simulink model "Project2FinalModel"  (R2024b)
settings: Solver=VariableStepAuto  StartTime=0.0  StopTime=300  RelTol=1e-3
values from neighbouring files (symbols this model uses):
  ca_f = 60000    [Project2Week1.m]
  ca_r = 90000    [Project2Week1.m]
  omega0 = 0    [Project2Week1.m]
  psi0 = 0    [Project2Week1.m]
  R = 200    [Project2Week1.m]
  vin = 2500    [Project2Week1.m]
  vlf = 1.25    [Project2Week1.m]
  vlr = vwbase - vlf    (= 1.25)    [Project2Week1.m]
  vmass = 1500    [Project2Week1.m]
  vwbase = 2.5    [Project2Week1.m]
  vy0 = 0    [Project2Week1.m]
  X0 = 0    [Project2Week1.m]
  Xd_simulink = [t_waypoints, Xd']    [Project2Week1.m]
  Y0 = 0    [Project2Week1.m]
  Yd_simulink = [t_waypoints, Yd']    [Project2Week1.m]
settings Model: Creator=btagl  LastModifiedBy=btagl

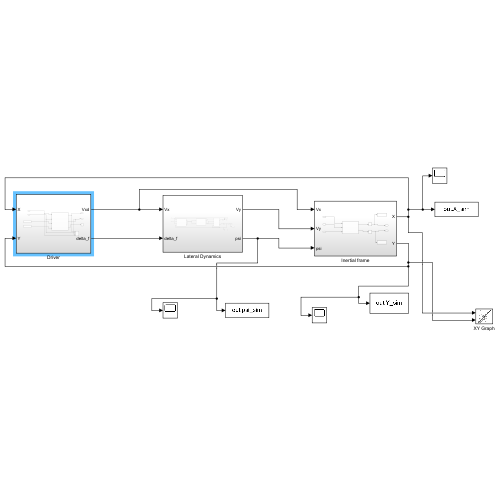
[thumbnail: Simulink's stored preview of the top-level diagram]
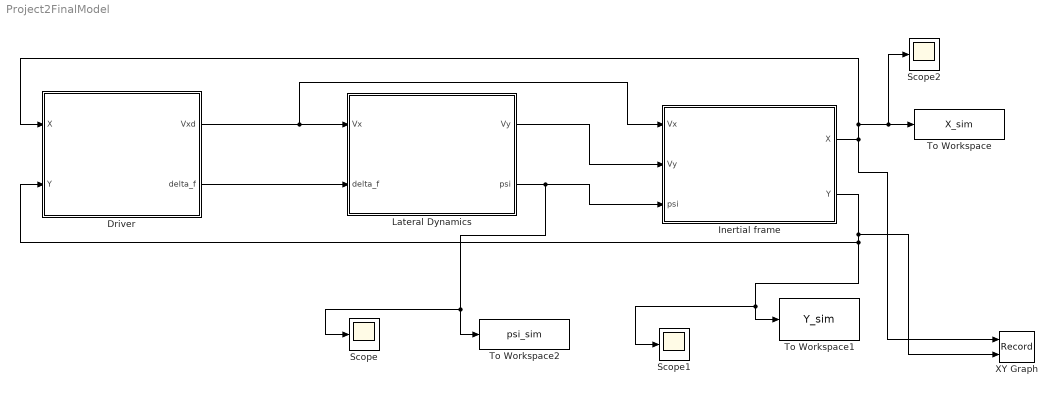
== system Project2FinalModel ==
  Driver : Subsystem
  Inertial frame : Subsystem
  Lateral Dynamics : Subsystem
  Scope : Scope
  Scope1 : Scope
  Scope2 : Scope
  To Workspace : ToWorkspace  VariableName=X_sim  SampleTime=-1
      settings: Save2DSignal=2-D array (concatenate along first dimension)
  To Workspace1 : ToWorkspace  VariableName=Y_sim  SampleTime=-1
      settings: Save2DSignal=2-D array (concatenate along first dimension)
  To Workspace2 : ToWorkspace  VariableName=psi_sim  SampleTime=-1
      settings: Save2DSignal=2-D array (concatenate along first dimension)
  XY Graph : Record  FileSettingsInternal="{\"entries\":[{\"content\":{\"excelSettings\":{\"content\":{},\"type\":\"Streamout.ExcelSettings\"}},\"type\":\"Streamout.FileSettingStorage\",\"uuid\":\"\"}],\"packageUris\":[\"http:\\/\\/schema.mathworks.com\\/mf0\\/streamout_blocks\\/R2020a\"],\"version\":\"1.0\"}"  Layout=[1 1]  SignalsInternal="{\"entries\":[{\"content\":{\"signals\":[{\"content\":{\"blockPath\":[],\"dimensions\":[1],\"domain\":\"\",\"lineColor\":\"#a2142f\",\"plots\":[ 1 ],\"port\":1,\"sid\":[\"\"],\"signalID\":1,\"signalName\":\"Inertial frame:1\"},\"type\":\"RecordBlkView.Signal\",\"uuid\":\"\"},{\"content\":{\"blockPath\":[],\"dimensions\":[1],\"domain\":\"\",\"lineColor\":\"#139fff\",\"plots\":[ 1 ],\"port\":2,\"sid\":[\"\"],\"signalID\":2,\"signalName\":\"Inertial frame:2\"},\"type\":\"RecordBlkView.Signal\",\"uuid\":\"\"}]},\"type\":\"RecordBlkView.InputSignals\",\"uuid\":\"\"}],\"packageUris\":[\"http:\\/\\/schema.mathworks.com\\/mf0\\/streamout_blocks\\/R2020a\"],\"version\":\"1.0\"}"  VisualizationBindings="{\"xyplotplugin\":{\"info\":[{\"series\":[{\"bindingParametersList\":[{\"parameter\":\"X-Axis\",\"signalID\":1,\"signalName\":\"Inertial frame:1\"},{\"parameter\":\"Y-Axis\",\"signalID\":2,\"signalName\":\"Inertial frame:2\"}],\"seriesID\":0}],\"subplotID\":1}]}}"  CompatibilityTag=XY
  wires:
  Driver/1(Vxd) -> Inertial frame/1(Vx), Lateral Dynamics/1(Vx)
  Driver/2(delta_f) -> Lateral Dynamics/2(delta_f)
  Inertial frame/2(Y) -> Scope1/1, To Workspace1/1, Driver/2(Y), XY Graph/2
  Lateral Dynamics/1(Vy) -> Inertial frame/2(Vy)
  Lateral Dynamics/2(psi) -> Scope/1, To Workspace2/1, Inertial frame/3(psi)
  Inertial frame/1(X) -> Scope2/1, To Workspace/1, Driver/1(X), XY Graph/1

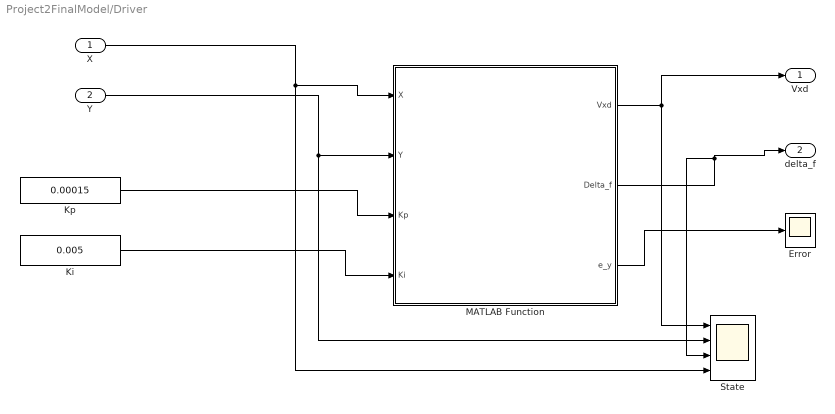
== system Project2FinalModel/Driver ==
  X : Inport
  Y : Inport  Port=2
  Error : Scope
  Ki : Constant  Value=0.005
  Kp : Constant  Value=0.00015
  MATLAB Function : MATLAB Function  TreatAsAtomicUnit=on
  State : Scope  NumInputPorts=4
  Vxd : Outport
  delta_f : Outport  Port=2
  wires:
  X/1 -> State/4, MATLAB Function/1(X)
  Y/1 -> State/2, MATLAB Function/2(Y)
  MATLAB Function/2(Delta_f) -> delta_f/1, State/3
  MATLAB Function/3(e_y) -> Error/1
  MATLAB Function/1(Vxd) -> Vxd/1, State/1
  Ki/1 -> MATLAB Function/4(Ki)
  Kp/1 -> MATLAB Function/3(Kp)

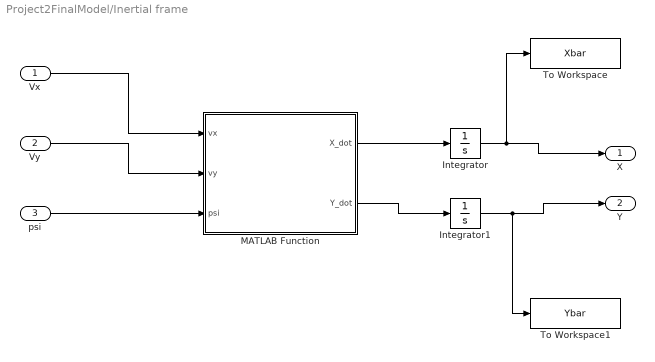
== system Project2FinalModel/Inertial frame ==
  Vx : Inport
  Vy : Inport  Port=2
  psi : Inport  Port=3
  Integrator : Integrator  InitialCondition=X0
  Integrator1 : Integrator  InitialCondition=Y0
  MATLAB Function : MATLAB Function  TreatAsAtomicUnit=on
  To Workspace : ToWorkspace  VariableName=Xbar  SampleTime=-1
      settings: Save2DSignal=2-D array (concatenate along first dimension)
  To Workspace1 : ToWorkspace  VariableName=Ybar  SampleTime=-1
      settings: Save2DSignal=2-D array (concatenate along first dimension)
  X : Outport
  Y : Outport  Port=2
  wires:
  MATLAB Function/2(Y_dot) -> Integrator1/1
  MATLAB Function/1(X_dot) -> Integrator/1
  Integrator/1 -> To Workspace/1, X/1
  Integrator1/1 -> To Workspace1/1, Y/1
  Vx/1 -> MATLAB Function/1(vx)
  Vy/1 -> MATLAB Function/2(vy)
  psi/1 -> MATLAB Function/3(psi)

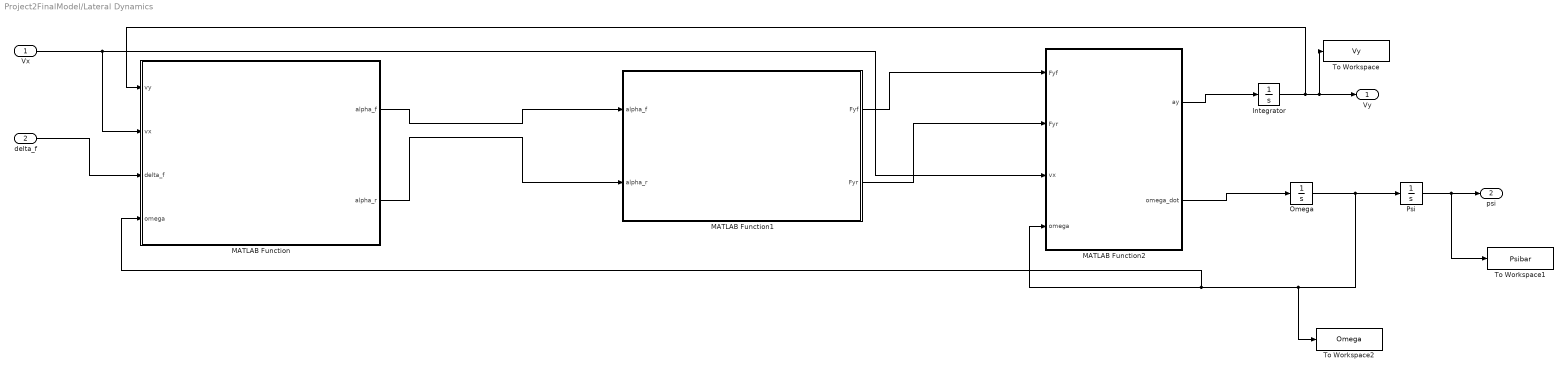
== system Project2FinalModel/Lateral Dynamics ==
  Vx : Inport
  delta_f : Inport  Port=2
  Integrator : Integrator  InitialCondition=vy0
  MATLAB Function : MATLAB Function  TreatAsAtomicUnit=on
  MATLAB Function1 : MATLAB Function  TreatAsAtomicUnit=on
  MATLAB Function2 : MATLAB Function  TreatAsAtomicUnit=on
  Omega : Integrator  InitialCondition=omega0
  Psi : Integrator  InitialCondition=psi0
  To Workspace : ToWorkspace  VariableName=Vy  SaveFormat=Timeseries  SampleTime=-1
  To Workspace1 : ToWorkspace  VariableName=Psibar  SampleTime=-1
  To Workspace2 : ToWorkspace  VariableName=Omega  SaveFormat=Timeseries  SampleTime=-1
  Vy : Outport
  psi : Outport  Port=2
  wires:
  Vx/1 -> MATLAB Function2/3(vx), MATLAB Function/2(vx)
  delta_f/1 -> MATLAB Function/3(delta_f)
  MATLAB Function/1(alpha_f) -> MATLAB Function1/1(alpha_f)
  MATLAB Function/2(alpha_r) -> MATLAB Function1/2(alpha_r)
  MATLAB Function1/1(Fyf) -> MATLAB Function2/1(Fyf)
  MATLAB Function1/2(Fyr) -> MATLAB Function2/2(Fyr)
  MATLAB Function2/2(omega_dot) -> Omega/1
  Omega/1 -> To Workspace2/1, MATLAB Function/4(omega), MATLAB Function2/4(omega), Psi/1
  MATLAB Function2/1(ay) -> Integrator/1
  Psi/1 -> To Workspace1/1, psi/1
  Integrator/1 -> MATLAB Function/1(vy), To Workspace/1, Vy/1

== matlab function Project2FinalModel/Lateral Dynamics/MATLAB Function ==
  data: vy input; alpha_f output; vx input; delta_f input; omega input; alpha_r output; vlf parameter; vlr parameter
function [alpha_f, alpha_r] = ComputeSlipAngles(vy, vx, delta_f, omega, vlf, vlr)
% Computes front and rear tire slip angles for a bicycle model

% Avoid division by zero if vx is very small
if abs(vx) < 0.01
    vx = 0.01; % Small positive velocity to prevent errors
end

% Compute front and rear slip angles
alpha_f = delta_f - atan((vy + vlf * omega) / vx);
alpha_r = -atan((vy - vlr * omega) / vx);
end

== matlab function Project2FinalModel/Driver/MATLAB Function ==
  settings: updateMethod=DISCRETE
  data: X input; Vxd output; Y input; Xd_simulink parameter; Yd_simulink parameter; R parameter; vwbase parameter; Delta_f output; Kp input; Ki input; e_y output
function [Vxd, Delta_f, e_y] = DriverPID(X, Y, Xd_simulink, Yd_simulink, R, vwbase, Kp, Ki)
Vxd = 15;  % m/s (constant speed)
% Persistent variables for integral term
persistent integral_error dt;
if isempty(integral_error)
   integral_error = 0;
   dt = 0.01;  % Simulation time step
end
% Extract waypoints
Xd = Xd_simulink(:, 2);
Yd = Yd_simulink(:, 2);
% Compute distances to waypoints
distances = sqrt((Xd - X).^2 + (Yd - Y).^2);
[~, idx] = min(distances);  % Find closest waypoint
% Look ahead a few waypoints for smoother control
lookahead_steps = 1;  % Number of waypoints to look ahead
lookahead_idx = min(idx + lookahead_steps, length(Yd));
% Compute nominal steering based on curvature
if Yd(lookahead_idx) == 0 || Yd(lookahead_idx) == 2 * R  % Car is on a straight
   Delta_f_base = 0;  % No steering needed
else
   Delta_f_base = atan(vwbase / R);  % Steering angle for the curve
end
% Compute Lateral Error using Lookahead (Y deviation from track center)
e_y = Yd(lookahead_idx) - Y; 
% Update integral error
integral_error = integral_error + e_y * dt;
% Compute Correction Term
Delta_f_correction = Kp * e_y + Ki * integral_error;
% Final Steering Command
Delta_f = Delta_f_base + Delta_f_correction;
end

== matlab function Project2FinalModel/Lateral Dynamics/MATLAB Function1 ==
  data: alpha_f input; Fyf output; alpha_r input; Fyr output; ca_f parameter; ca_r parameter
function [Fyf, Fyr] = ComputeTireForces(alpha_f, alpha_r, ca_f, ca_r)
% Computes front and rear lateral tire forces using linear tire model

% Compute lateral forces
Fyf = ca_f * alpha_f;
Fyr = ca_r * alpha_r;
end

== matlab function Project2FinalModel/Lateral Dynamics/MATLAB Function2 ==
  data: Fyf input; ay output; Fyr input; vx input; omega input; omega_dot output; vmass parameter; vlf parameter; vlr parameter; vin parameter
function [ay, omega_dot] = LateralDynamics(Fyf, Fyr, vx, omega, vmass, vlf, vlr, vin)
% Computes lateral acceleration (ay) and yaw acceleration (omega_dot)
% for a simple bicycle model.

% Compute Lateral Acceleration
Fy = Fyf + Fyr;
ay = Fy / vmass - omega * vx;

% Compute Yaw Acceleration
M = Fyf * vlf - Fyr * vlr;
omega_dot = M / vin;
end

== matlab function Project2FinalModel/Inertial frame/MATLAB Function ==
  data: vx input; X_dot output; vy input; psi input; Y_dot output
function [X_dot, Y_dot] = KinematicsInertial(vx, vy, psi)
% Converts body-frame velocity (vx, vy) into global coordinates (X, Y)

% Compute global velocity components
X_dot = vx * cos(psi) - vy * sin(psi);
Y_dot = vx * sin(psi) + vy * cos(psi);

end
